simulink model "DC_control_harness"  (R2023b)
settings: Solver=FixedStepAuto  StartTime=0.0  StopTime=inf  FixedStep=2.6667e-04  RelTol=1e-4  AbsTol=1e-6
settings Model: DataDictionary=fmuGenerationDictionay.sldd  ModifiedByFormat=Third Equation Ltd  Creator=Third Equation Ltd  LastModifiedBy=Third Equation Ltd
settings ConfigSet: Description=|
  | Reference configuration for protected model and FMU generation
  | Sample frequency = 3750 Hz
settings SolverCC: AutoScaleAbsTol=off  AlgebraicLoopSolver=TrustRegion  MaxZcPerStep=1
settings DataIOCC: ExternalInput=[]  InitialState=[]  SaveFormat=Array  SaveOutput=off  SaveTime=off  ReturnWorkspaceOutputs=off
settings OptimizationCC: BlockReduction=off  BooleanDataType=off  ReuseModelBlockBuffer=off  ExpressionDepthLimit=2147483647  InitFltsAndDblsToZero=on
settings DebuggingCC: SaveWithParameterizedLinksMsg=none  SignalResolutionControl=TryResolveAllWithWarning  MultiTaskDSMMsg=warning  MultiTaskCondExecSysMsg=none  IntegerOverflowMsg=none  FcnCallInpInsideContextMsg=warning  UnconnectedInputMsg=warning  UnconnectedOutputMsg=warning  UnconnectedLineMsg=warning  StateNameClashWarn=warning  SFUnexpectedBacktrackingDiag=warning  SFNoUnconditionalDefaultTransitionDiag=warning  SFExecutionAtInitializationDiag=none  IntegerSaturationMsg=none  UnderSpecifiedDimensionMsg=warning  ArithmeticOperatorsInVariantConditions=warning
settings HardwareCC: ProdBitPerPointer=32  ProdBitPerSizeT=32  ProdBitPerPtrDiffT=32  ProdLargestAtomicFloat=None  ProdWordSize=32  ProdHWDeviceType=Custom Processor->Custom Processor
settings ModelReferenceCC: EnableRefExpFcnMdlSchedulingChecks=on  PropagateSignalLabelsOutOfModel=off
settings SFSimCC: SimUseLocalCustomCode=off  CustomCodeUndefinedFunction=UseInterfaceOnly
settings RTWCC: Description=FMU2CS  SystemTargetFile=fmu2cs.tlc  TemplateMakefile=fmu2cs_default_tmf  RTWUseLocalCustomCode=off  DLArmComputeVersion=19.05
settings CodeAppCC: StateflowObjectComments=on
settings GRTTargetCC: TargetLangStandard=C89/C90 (ANSI)  CombineOutputUpdateFcns=off  MatFileLogging=off
settings ConfigComp: CovMetricSettings=dw  CovSaveCumulativeToWorkspaceVar=on  CovSaveSingleToWorkspaceVar=on  CovExternalEMLEnable=off  CovSFcnEnable=off

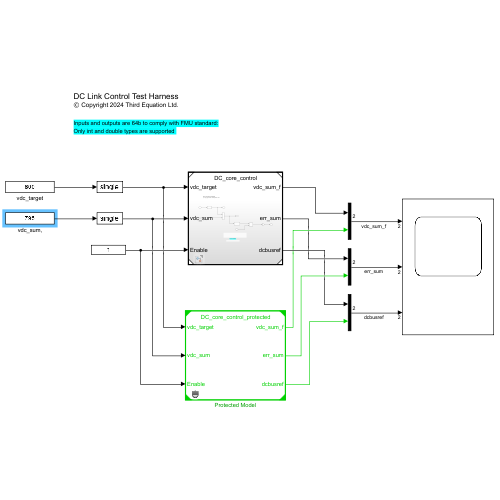
[thumbnail: Simulink's stored preview of the top-level diagram]
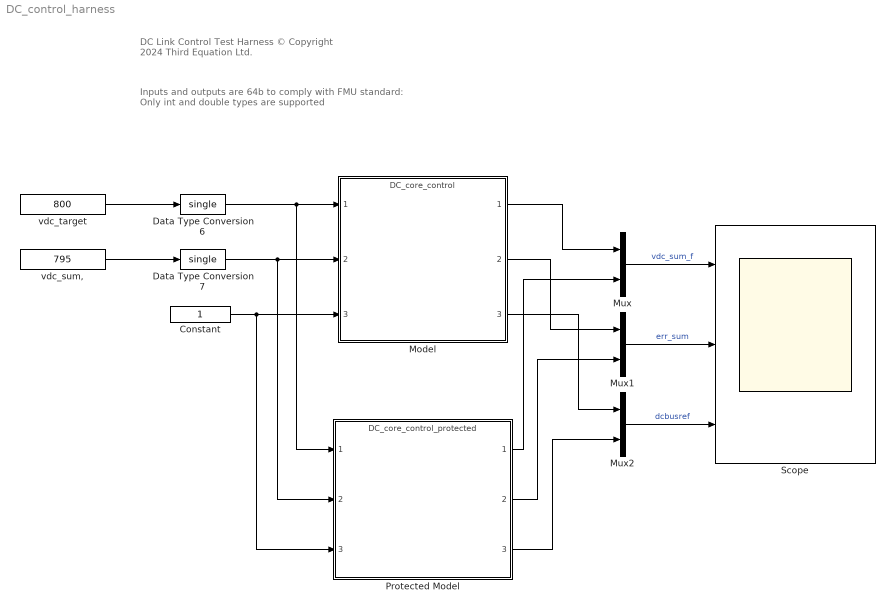
== system DC_control_harness ==
  note: Inputs and outputs are 64b to comply with FMU standard:
      | Only int and double types are supported
  note: DC Link Control Test Harness
      | © Copyright 2024 Third Equation Ltd.
  Constant : Constant  OutDataTypeStr=boolean
  Data Type Conversion6 : DataTypeConversion  OutDataTypeStr=single  SaturateOnIntegerOverflow=off  RndMeth=Floor
  Data Type Conversion7 : DataTypeConversion  OutDataTypeStr=single  SaturateOnIntegerOverflow=off  RndMeth=Floor
  Model : ModelReference  ModelNameDialog=DC_core_control.slx  SimulationMode=Normal  ModelReferenceVersion=1.16
  Mux : Mux  Inputs=2
  Mux1 : Mux  Inputs=2
  Mux2 : Mux  Inputs=2
  Protected Model : ModelReference  ModelNameDialog=DC_core_control_protected.slxp  ModelReferenceVersion=1.16  CopyOfModelProtected=on
  Scope : Scope  NumInputPorts=3
  vdc_sum, : Constant  Value=795  OutDataTypeStr=double
  vdc_target : Constant  Value=800  OutDataTypeStr=double
  wires:
  Constant/1 -> Model/3, Protected Model/3
  Data Type Conversion6/1 -> Model/1, Protected Model/1
  vdc_target/1 -> Data Type Conversion6/1
  Data Type Conversion7/1 -> Model/2, Protected Model/2
  vdc_sum,/1 -> Data Type Conversion7/1
  Model/1 -> Mux/1
  Model/2 -> Mux1/1
  Model/3 -> Mux2/1
  Mux/1 -> Scope/1  "vdc_sum_f"
  Mux1/1 -> Scope/2  "err_sum"
  Mux2/1 -> Scope/3  "dcbusref"
  Protected Model/1 -> Mux/2
  Protected Model/2 -> Mux1/2
  Protected Model/3 -> Mux2/2
